simulink model "backup"  (R2019b)
settings: Solver=ode1  StartTime=0.0  StopTime=Inf  FixedStep=0.001  RelTol=1e-3
PostLoadFcn:
  | , if any(exist('dsrtsu_mdlpostloadfcn', 'file') ~= 0), dsrtsu_mdlpostloadfcn('Execute', bdroot); end,
InitFcn:
  | , if any(exist('dsmpb_private', 'file') ~= 0), dsmpb_private('dsmpb_mdlclblib', 'Init', bdroot); end,
libraries: VSIGenLib x5, dsmpblib x5, etargetslib x1
PreSaveFcn:
  | , if any(exist('dsmpb_private', 'file') ~= 0), dsmpb_private('dsmpb_mdlclblib', 'PreSave', bdroot); end,
CloseFcn:
  | , if any(exist('dsmpb_private', 'file') ~= 0), dsmpb_private('dsmpb_mdlclblib', 'Close', bdroot); end,
Description:
  | Standard RTI1006 template.
  | Supported MATLAB version:  R2019b.
settings Model: Tag=RTI1006  DSRTSU_INTERNAL_RTI_VER=550  DSRTSU_INTERNAL_RTI_TYPE=rti1006  RTICANMMDATA=struct('GeneralSetupData',struct('modelroot','C:\GitDev\Anye','generalsettings',struct('filesettings',struct('destfolder',struct('Name','RTICANMM_FILES','Check',1),'buildfolder',struct('Name','.','Check',1),'AbsDestfolder',struct('Name','C:\GitDev\Anye\RTICANMM_FILES'),'AbsBuildfolder',struct('Name','C:\GitDev\Anye'))),'options',struct('addpaths',1,'rmpaths',1,'addtrcexclusion',true,'cannavigator',struct('checkmonitoring',0),'show_usrtrc',0,'use_usrtrc',0),'advanced',struct('options',ones(1,100)),'MPSetup',{{}},'RTI',struct('Type','RTI1006','Ver','7.13','Date','02-Nov-2019'),'modelname','','block','untitled'))  DSRTSU_INTERNAL_RTIFPGA=150  DSMPB_ID_DATA={'27',struct('BlockId','67fb374a-304a-478f-a592-1aee3a505a2b','SignalIds',{{'2d54aa05-414c-4825-8c9f-0988bd06d144','536830b0-e070-4266-9be7-997bb7b1e681','e70da20a-ea0d-44d6-b900-eb8aacf6428a','20288d3c-8621-4fce-9468-03dd559dfda3'}}),'29',struct('BlockId','0dbda633-5747-40ab-98bf-a324bbe7dd23','SignalIds',{{'0685f9a0-0925-49db-ab70-ff46489f5fe8','33715b38-3a7a-4218-8ad6-97abd4ab1f54'}}),'30',struct('BlockId','6ab39375-0e3b-4637-a550-6a5a64ee5535','SignalIds',{{'045dec7c-803b-4cce-9d63-4ff7dc08015a'}}),'35',struct('BlockId','1b8d31d4-cea8-4f71-9209-0764cd46e912','SignalIds',{{'f6ec3d0e-8074-4a92-b6d9-d000939805f9','03552e9d-9230-4b4f-a700-49d1c2ef293c'}}),'36',struct('BlockId','ecaf8e8d-8e5b-4759-9d99-8e442d2e6bba','SignalIds',{{'6a45647f-2bfe-414a-817f-b96e9d7edfb2'}})}  Creator=RVDP  LastModifiedBy=RVDP
settings DataIOCC: ReturnWorkspaceOutputs=off
settings OptimizationCC: BlockReduction=off  OptimizeBlockIOStorage=off  BufferReuse=off  GlobalBufferReuse=off  ExpressionFolding=off  LocalBlockOutputs=off  OptimizeDataStoreBuffers=off  BusAssignmentInplaceUpdate=off
settings DebuggingCC: PregeneratedLibrarySubsystemCodeDiagnostic=none  ArithmeticOperatorsInVariantConditions=warning
settings HardwareCC: ProdBitPerPointer=32  ProdBitPerSizeT=32  ProdBitPerPtrDiffT=32  ProdLargestAtomicInteger=Integer  ProdWordSize=32  ProdHWDeviceType=Custom Processor->Custom  TargetIntDivRoundTo=Zero  TargetEndianess=LittleEndian  TargetHWDeviceType=Custom Processor->Custom
settings SFSimCC: SimUseLocalCustomCode=off  MATLABDynamicMemAlloc=off  CustomCodeUndefinedFunction=UseInterfaceOnly
settings RTWCC: Description=dSPACE DS1006 Hardware Platform  SystemTargetFile=rti1006.tlc  MakeCommand=make_rti  TemplateMakefile=rti1006.tmf  RTWUseLocalCustomCode=off
settings CodeAppCC: StateflowObjectComments=on
settings STFCustomTargetCC: ParMdlRefBuildCompliant=on  MatFileLogging=on  SystemTargetFile=rti1006.tlc
settings GRTTargetCC: TargetLangStandard=C89/C90 (ANSI)  CompOptLevelCompliant=off  ConcurrentExecutionCompliant=off  CombineOutputUpdateFcns=off  CPPClassGenCompliant=off  UseToolchainInfoCompliant=off
settings ConfigComp: CovMetricSettings=dswe

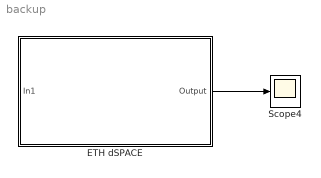
== system backup ==
  ETH dSPACE : Subsystem
  Scope4 : Scope
  wires:
  ETH dSPACE/1(Output) -> Scope4/1
  ? -> ETH dSPACE/1(In1)

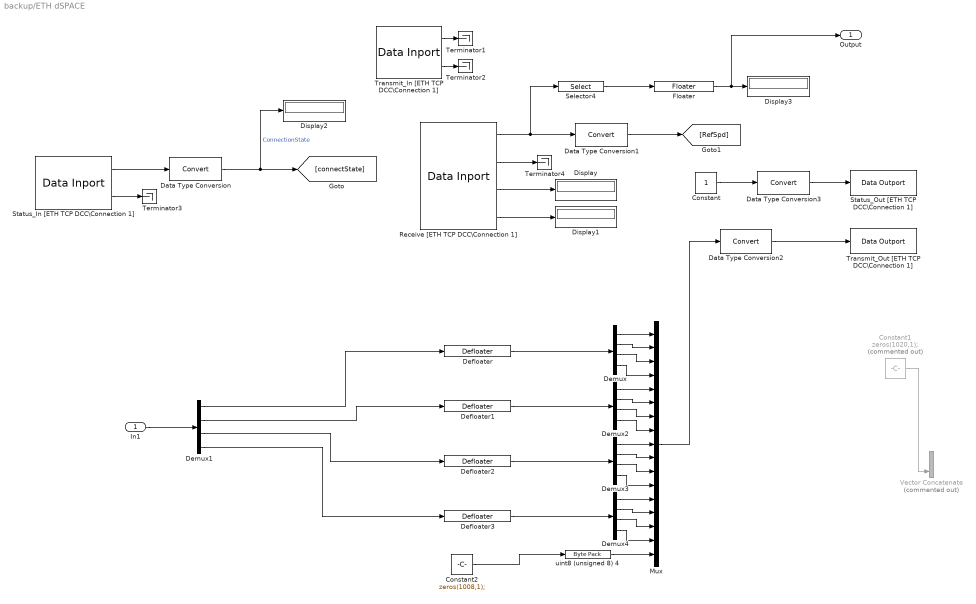
== system backup/ETH dSPACE ==
  In1 : Inport
  Constant : Constant
  Constant1 : Constant  Commented=on  Value=zeros(1020,1);
  Constant2 : Constant  Value=zeros(1008,1);  OutDataTypeStr=uint8
  Data Type Conversion{,1..3} (4 alike) : DataTypeConversion
  Defloater{,1..3} (4 alike) : VSIGenLib/Defloater  SystemSampleTime=-1  Latency=0  AutoFrameSizeCalculation=off
  Demux{,1..4} (5 alike) : Demux
  Display{,1..3} (4 alike) : Display
  Floater : VSIGenLib/Floater  SystemSampleTime=-1  Latency=0  AutoFrameSizeCalculation=off
  Mux : Mux  Inputs=17
  Receive [ETH TCP DCC\Connection 1] : dsmpblib/Data Inport  Priority=10000
      settings: SourceProductName=dSPACE Model Interface Blockset
  Selector4 : Selector  IndexMode=Zero-based  InputPortWidth=1024  IndexOptions=Index vector (dialog)  Indices=[1 2 3 4]  OutputSizes=1
  Status_In [ETH TCP DCC\Connection 1] : dsmpblib/Data Inport  Priority=10000
      settings: SourceProductName=dSPACE Model Interface Blockset
  Status_Out [ETH TCP DCC\Connection 1] : dsmpblib/Data Outport  Priority=-10000
      settings: SourceProductName=dSPACE Model Interface Blockset
  Terminator{1..4} (4 alike) : Terminator
  Transmit_In [ETH TCP DCC\Connection 1] : dsmpblib/Data Inport  Priority=10000
      settings: SourceProductName=dSPACE Model Interface Blockset
  Transmit_Out [ETH TCP DCC\Connection 1] : dsmpblib/Data Outport  Priority=-10000
      settings: SourceProductName=dSPACE Model Interface Blockset
  Vector Concatenate : Concatenate  Commented=on
  uint8 (unsigned 8) 4 : etargetslib/Byte Pack  datatypes={'uint8'}  byteAlign=1
      settings: SourceProductName=MATLAB Coder
  Output : Outport
  wires:
  Transmit_In [ETH TCP DCC\Connection 1]/1 -> Terminator1/1
  Data Type Conversion1/1 -> [RefSpd]
  Data Type Conversion2/1 -> Transmit_Out [ETH TCP DCC\Connection 1]/1
  Constant1/1 -> Vector Concatenate/2
  Receive [ETH TCP DCC\Connection 1]/1 -> Selector4/1, Data Type Conversion1/1
  Status_In [ETH TCP DCC\Connection 1]/2 -> Terminator3/1
  Selector4/1 -> Floater/1
  Data Type Conversion3/1 -> Status_Out [ETH TCP DCC\Connection 1]/1
  Data Type Conversion/1 -> Display2/1, [connectState]  "ConnectionState"
  Receive [ETH TCP DCC\Connection 1]/2 -> Terminator4/1
  Floater/1 -> Output/1, Display3/1
  Receive [ETH TCP DCC\Connection 1]/3 -> Display/1
  Receive [ETH TCP DCC\Connection 1]/4 -> Display1/1
  Transmit_In [ETH TCP DCC\Connection 1]/2 -> Terminator2/1
  Status_In [ETH TCP DCC\Connection 1]/1 -> Data Type Conversion/1
  Constant/1 -> Data Type Conversion3/1
  Defloater/1 -> Demux/1
  In1/1 -> Demux1/1
  Demux1/1 -> Defloater/1
  Defloater1/1 -> Demux2/1
  Defloater2/1 -> Demux3/1
  Defloater3/1 -> Demux4/1
  Demux1/2 -> Defloater1/1
  Demux1/3 -> Defloater2/1
  Demux1/4 -> Defloater3/1
  Constant2/1 -> uint8 (unsigned 8) 4/1
  Demux/1 -> Mux/1
  Demux/2 -> Mux/2
  Demux/3 -> Mux/3
  Demux/4 -> Mux/4
  Demux2/1 -> Mux/5
  Demux2/2 -> Mux/6
  Demux2/3 -> Mux/7
  Demux2/4 -> Mux/8
  Demux3/1 -> Mux/9
  Demux3/2 -> Mux/10
  Demux3/3 -> Mux/11
  Demux3/4 -> Mux/12
  Demux4/1 -> Mux/13
  Demux4/2 -> Mux/14
  Demux4/3 -> Mux/15
  Demux4/4 -> Mux/16
  uint8 (unsigned 8) 4/1 -> Mux/17
  Mux/1 -> Data Type Conversion2/1
